simulink model "Simulation_Block_Diagram_Performance"  (R2015b)
settings: Solver=ode1  StartTime=0.0  StopTime=1200  FixedStep=0.1  RelTol=1e-3
undefined symbols (not defined in the file): udds
settings Model: Creator=wasynczu  LastModifiedBy=Kane Chew
settings DataIOCC: LimitDataPoints=off
settings DebuggingCC: ParameterUnderflowMsg=error

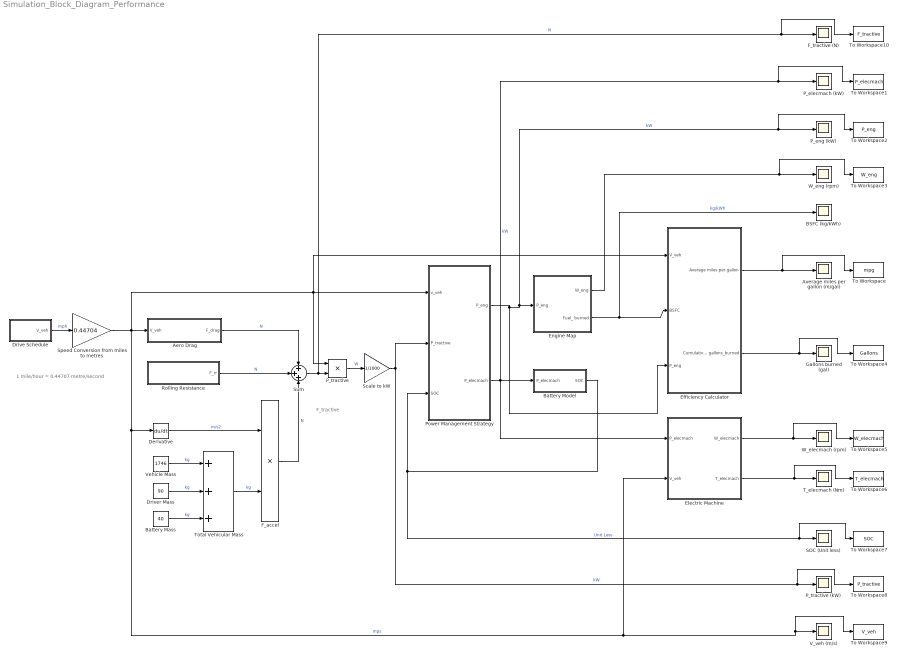
== system Simulation_Block_Diagram_Performance ==
  note: F_tractive
  note: 1 mile/hour = 0.44707 metre/second
  Aero Drag : Subsystem
  Average miles per gallon (m/gal) : Scope
  BSFC (kg/kWh) : Scope
  Battery Mass : Constant  Value=40
  "Battery Model " : Subsystem
  Derivative : Derivative
  "Drive Schedule " : Subsystem
  Driver Mass : Constant  Value=90
  Efficiency Calculator : Subsystem
  Electric Machine : Subsystem
  Engine Map : Subsystem
  F_accel : Product
  F_tractive (N) : Scope
  Gallons burned (gal) : Scope
  P_elecmach (kW) : Scope
  P_eng (kW) : Scope
  P_tractive : Product  Inputs=**
  P_tractive (kW) : Scope
  Power Management Strategy : MATLAB Function  TreatAsAtomicUnit=on
  Rolling Resistance : Subsystem
  SOC (Unit less) : Scope
  Scale to kW : Gain  Gain=1/1000
  Speed Conversion from miles to metres : Gain  Gain=0.44704
  Sum : Sum  Inputs=+++
  T_elecmach (Nm) : Scope
  To Workspace : ToWorkspace  VariableName=mpg  SaveFormat=Timeseries  SampleTime=-1
  To Workspace1 : ToWorkspace  VariableName=P_elecmach  SaveFormat=Timeseries  SampleTime=-1
  To Workspace10 : ToWorkspace  VariableName=F_tractive  SaveFormat=Timeseries  SampleTime=-1
  To Workspace2 : ToWorkspace  VariableName=P_eng  SaveFormat=Timeseries  SampleTime=-1
  To Workspace3 : ToWorkspace  VariableName=W_eng  SaveFormat=Timeseries  SampleTime=-1
  To Workspace4 : ToWorkspace  VariableName=Gallons  SaveFormat=Timeseries  SampleTime=-1
  To Workspace5 : ToWorkspace  VariableName=W_elecmach  SaveFormat=Timeseries  SampleTime=-1
  To Workspace6 : ToWorkspace  VariableName=T_elecmach  SaveFormat=Timeseries  SampleTime=-1
  To Workspace7 : ToWorkspace  VariableName=SOC  SaveFormat=Timeseries  SampleTime=-1
  To Workspace8 : ToWorkspace  VariableName=P_tractive  SaveFormat=Timeseries  SampleTime=-1
  To Workspace9 : ToWorkspace  VariableName=V_veh  SaveFormat=Timeseries  SampleTime=-1
  Total Vehicular Mass : Sum  Inputs=+++
  V_veh (m/s) : Scope
  Vehicle Mass : Constant  Value=1746
  W_elecmach (rpm) : Scope
  "W_eng (rpm) " : Scope
  wires:
  Speed Conversion from miles to metres/1 -> Electric Machine/2("V_veh "), To Workspace9/1, V_veh (m/s)/1, Derivative/1, Efficiency Calculator/1("V_veh "), Power Management Strategy/1(v_veh), P_tractive/1, Aero Drag/1(V_veh)  "mps"
  Derivative/1 -> F_accel/1  "m/s2"
  Aero Drag/1("F_drag ") -> Sum/1  "N"
  Rolling Resistance/1("F_rr ") -> Sum/2  "N"
  Sum/1 -> To Workspace10/1, F_tractive (N)/1, P_tractive/2  "N"
  P_tractive/1 -> Scale to kW/1  "W"
  Power Management Strategy/1(P_eng) -> Efficiency Calculator/3("P_eng "), To Workspace2/1, P_eng (kW)/1, Engine Map/1(P_eng)  "kW"
  "Drive Schedule "/1("V_veh ") -> Speed Conversion from miles to metres/1  "mph"
  Power Management Strategy/2(P_elecmach) -> Electric Machine/1(P_elecmach), To Workspace1/1, P_elecmach (kW)/1, "Battery Model "/1(P_elecmach)  "kW"
  "Battery Model "/1(SOC) -> Power Management Strategy/3(SOC), To Workspace7/1, SOC (Unit less)/1  "Unit Less"
  Engine Map/2(Fuel_ burned) -> BSFC (kg/kWh)/1, Efficiency Calculator/2(BSFC)  "kg/kWh"
  Engine Map/1(W_eng) -> To Workspace3/1, "W_eng (rpm) "/1
  Scale to kW/1 -> To Workspace8/1, P_tractive (kW)/1, Power Management Strategy/2(P_tractive)  "kW"
  Efficiency Calculator/1(Average miles per gallon) -> To Workspace/1, Average miles per gallon (m/gal)/1
  Efficiency Calculator/2(Cumulative gallons_burned) -> To Workspace4/1, Gallons burned (gal)/1
  Battery Mass/1 -> Total Vehicular Mass/3  "kg"
  Driver Mass/1 -> Total Vehicular Mass/2  "kg"
  Vehicle Mass/1 -> Total Vehicular Mass/1  "kg"
  Total Vehicular Mass/1 -> F_accel/2  "kg"
  F_accel/1 -> Sum/3  "N"
  Electric Machine/1(W_elecmach) -> To Workspace5/1, W_elecmach (rpm)/1
  Electric Machine/2(T_elecmach) -> To Workspace6/1, T_elecmach (Nm)/1

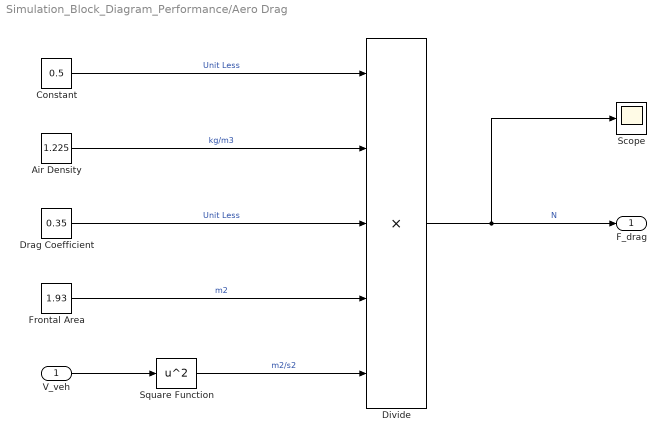
== system Simulation_Block_Diagram_Performance/Aero Drag ==
  V_veh : Inport
  Air Density : Constant  Value=1.225
  Constant : Constant  Value=0.5
  Divide : Product  Inputs=*****
  Drag Coefficient : Constant  Value=0.35
  Frontal Area : Constant  Value=1.93
  Scope : Scope
  Square Function : Math  Operator=square  SaturateOnIntegerOverflow=on
  "F_drag " : Outport
  wires:
  Divide/1 -> Scope/1, "F_drag "/1  "N"
  Air Density/1 -> Divide/2  "kg/m3"
  V_veh/1 -> Square Function/1
  Constant/1 -> Divide/1  "Unit Less"
  Frontal Area/1 -> Divide/4  "m2"
  Drag Coefficient/1 -> Divide/3  "Unit Less"
  Square Function/1 -> Divide/5  "m2/s2"

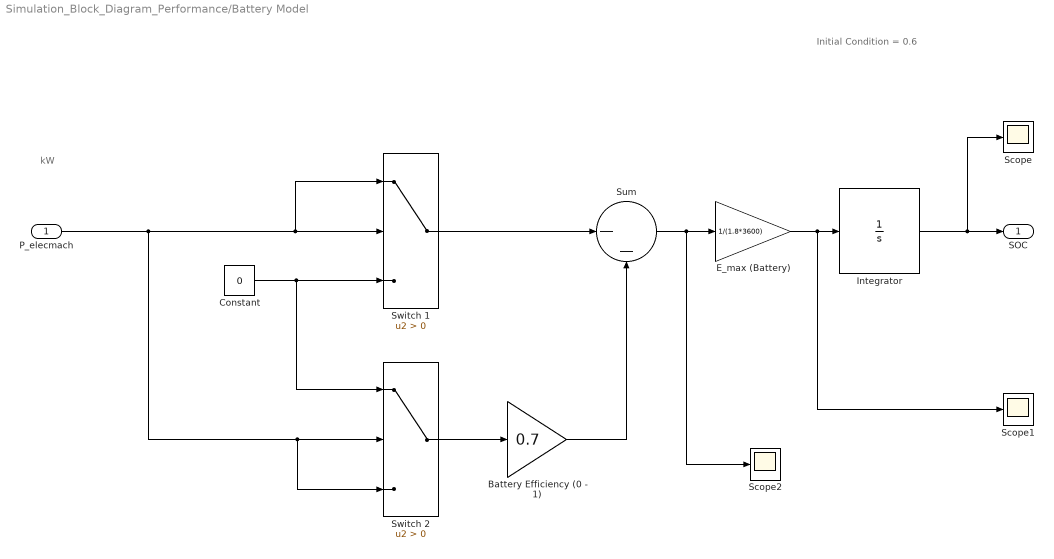
== system Simulation_Block_Diagram_Performance/Battery Model  ==
  note: kW
  note: Initial Condition = 0.6
  P_elecmach : Inport
  Battery Efficiency (0 - 1) : Gain  Gain=0.7
  Constant : Constant  Value=0
  E_max (Battery) : Gain  Gain=1/(1.8*3600)
  Integrator : Integrator  InitialCondition=0.6
  Scope : Scope
  Scope1 : Scope
  Scope2 : Scope
  Sum : Sum  Inputs=|--
  Switch 1 : Switch  Criteria=u2 > Threshold
  Switch 2 : Switch  Criteria=u2 > Threshold
  SOC : Outport
  wires:
  P_elecmach/1 -> Switch 2/3, Switch 2/2, Switch 1/1, Switch 1/2
  Constant/1 -> Switch 2/1, Switch 1/3
  Switch 1/1 -> Sum/1
  Switch 2/1 -> Battery Efficiency (0 - 1)/1
  Battery Efficiency (0 - 1)/1 -> Sum/2
  Sum/1 -> E_max (Battery)/1, Scope2/1
  E_max (Battery)/1 -> Scope1/1, Integrator/1
  Integrator/1 -> Scope/1, SOC/1

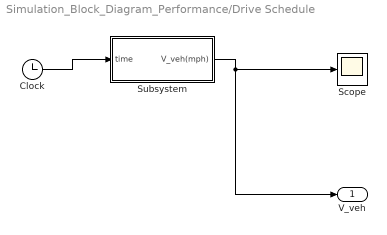
== system Simulation_Block_Diagram_Performance/Drive Schedule  ==
  Clock : Clock
  Scope : Scope
  Subsystem : Subsystem  mask{schedule=udds}
      mask prompts: schedule "drive schedule"
      mask init:
      | N=length(schedule(:,1))
  "V_veh " : Outport
  wires:
  Clock/1 -> Subsystem/1(time)
  Subsystem/1(V_veh(mph)) -> "V_veh "/1, Scope/1

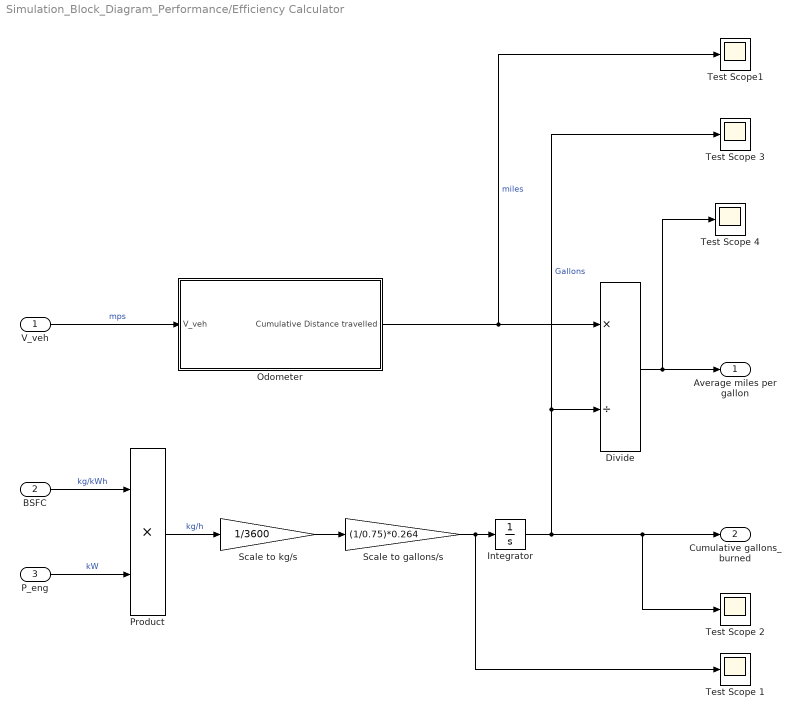
== system Simulation_Block_Diagram_Performance/Efficiency Calculator ==
  "V_veh " : Inport
  BSFC : Inport  Port=2
  "P_eng " : Inport  Port=3
  Divide : Product  Inputs=*/
  Integrator : Integrator  InitialCondition=0.001
  "Odometer " : Subsystem
  Product : Product
  Scale to gallons/s : Gain  Gain=(1/0.75)*0.264
  Scale to kg/s : Gain  Gain=1/3600
  Test Scope {1..4} (4 alike) : Scope
  Test Scope1 : Scope
  Average miles per gallon : Outport
  Cumulative gallons_burned : Outport  Port=2
  wires:
  Integrator/1 -> Divide/2, Test Scope 3/1, Test Scope 2/1, Cumulative gallons_burned/1  "Gallons"
  "V_veh "/1 -> "Odometer "/1(V_veh)  "mps"
  "Odometer "/1(Cumulative Distance travelled) -> Test Scope1/1, Divide/1  "miles"
  Divide/1 -> Test Scope 4/1, Average miles per gallon/1
  Product/1 -> Scale to kg/s/1  "kg/h"
  BSFC/1 -> Product/1  "kg/kWh"
  "P_eng "/1 -> Product/2  "kW"
  Scale to kg/s/1 -> Scale to gallons/s/1
  Scale to gallons/s/1 -> Test Scope 1/1, Integrator/1

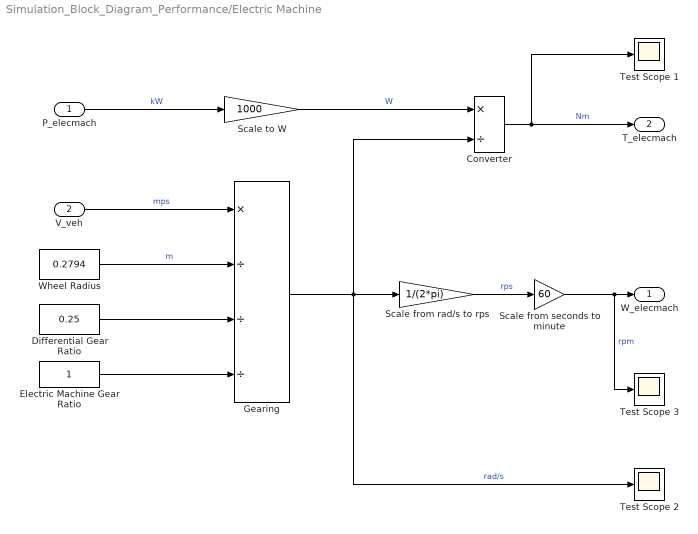
== system Simulation_Block_Diagram_Performance/Electric Machine ==
  P_elecmach : Inport
  "V_veh " : Inport  Port=2
  Converter : Product  Inputs=*/
  Differential Gear Ratio : Constant  Value=0.25
  Electric Machine Gear Ratio : Constant
  Gearing : Product  Inputs=*///
  Scale from rad/s to rps : Gain  Gain=1/(2*pi)
  Scale from seconds to minute : Gain  Gain=60
  Scale to W : Gain  Gain=1000
  Test Scope 1 : Scope
  Test Scope 2 : Scope
  Test Scope 3 : Scope
  Wheel Radius : Constant  Value=0.2794
  W_elecmach : Outport
  T_elecmach : Outport  Port=2
  wires:
  Gearing/1 -> Scale from rad/s to rps/1, Converter/2, Test Scope 2/1  "rad/s"
  Wheel Radius/1 -> Gearing/2  "m"
  Differential Gear Ratio/1 -> Gearing/3
  Electric Machine Gear Ratio/1 -> Gearing/4
  Converter/1 -> Test Scope 1/1, T_elecmach/1  "Nm"
  "V_veh "/1 -> Gearing/1  "mps"
  Scale from seconds to minute/1 -> Test Scope 3/1, W_elecmach/1  "rpm"
  P_elecmach/1 -> Scale to W/1  "kW"
  Scale to W/1 -> Converter/1  "W"
  Scale from rad/s to rps/1 -> Scale from seconds to minute/1  "rps"

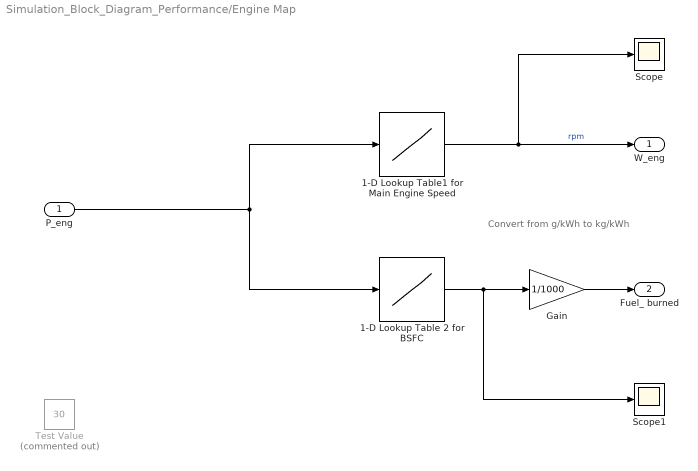
== system Simulation_Block_Diagram_Performance/Engine Map ==
  note: Convert from g/kWh to kg/kWh
  P_eng : Inport
  "1-D Lookup Table 2 for BSFC " : Lookup_n-D  NumberOfTableDimensions=1  BreakpointsForDimension1=[7,12,24,35,47,57,77,82,85]  BreakpointsForDimension2=[7,12,24,35,47]  Table=[500,400,320,285,265,255,255,265,285]  InternalRulePriority=Speed  RndMeth=Simplest  InputSameDT=on
  1-D Lookup Table1 for Main Engine Speed : Lookup_n-D  NumberOfTableDimensions=1  BreakpointsForDimension1=[7,12,24,35,47,57,77,82,85]  BreakpointsForDimension2=[7,12,24,35,47]  Table=[1009,1183,1588,1936,2318,2612,3371,3685,4014]  InternalRulePriority=Speed  RndMeth=Simplest  InputSameDT=on
  Gain : Gain  Gain=1/1000
  Scope : Scope
  Scope1 : Scope
  Test Value : Constant  Commented=on  Value=30
  W_eng : Outport
  Fuel_ burned : Outport  Port=2
  wires:
  1-D Lookup Table1 for Main Engine Speed/1 -> Scope/1, W_eng/1  "rpm"
  "1-D Lookup Table 2 for BSFC "/1 -> Scope1/1, Gain/1
  P_eng/1 -> "1-D Lookup Table 2 for BSFC "/1, 1-D Lookup Table1 for Main Engine Speed/1
  Gain/1 -> Fuel_ burned/1

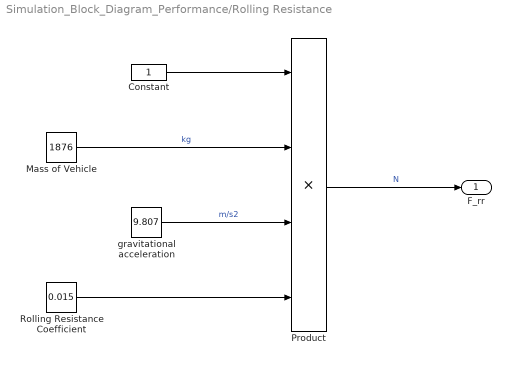
== system Simulation_Block_Diagram_Performance/Rolling Resistance ==
  Constant : Constant
  Mass of Vehicle : Constant  Value=1876
  "Product " : Product  Inputs=****
  Rolling Resistance Coefficient : Constant  Value=0.015
  "gravitational acceleration " : Constant  Value=9.807
  "F_rr " : Outport
  wires:
  Constant/1 -> "Product "/1
  "Product "/1 -> "F_rr "/1  "N"
  Mass of Vehicle/1 -> "Product "/2  "kg"
  Rolling Resistance Coefficient/1 -> "Product "/4
  "gravitational acceleration "/1 -> "Product "/3  "m/s2"

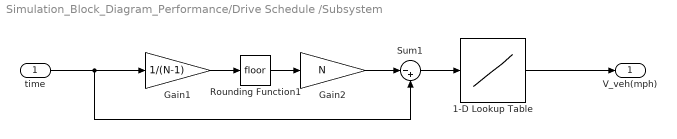
== system Simulation_Block_Diagram_Performance/Drive Schedule /Subsystem ==
  time : Inport
  1-D Lookup Table : Lookup_n-D  NumberOfTableDimensions=1  BreakpointsForDimension1=schedule(:,1)  Table=schedule(:,2)  InternalRulePriority=Speed  RndMeth=Simplest  InputSameDT=on
  Gain1 : Gain  Gain=1/(N-1)
  Gain2 : Gain  Gain=N
  Rounding Function1 : Rounding
  Sum1 : Sum  Inputs=|-+
  V_veh(mph) : Outport
  wires:
  Gain1/1 -> Rounding Function1/1
  Rounding Function1/1 -> Gain2/1
  Gain2/1 -> Sum1/1
  Sum1/1 -> 1-D Lookup Table/1
  time/1 -> Sum1/2, Gain1/1
  1-D Lookup Table/1 -> V_veh(mph)/1

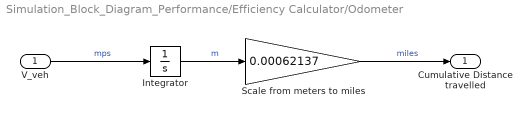
== system Simulation_Block_Diagram_Performance/Efficiency Calculator/Odometer  ==
  V_veh : Inport
  Integrator : Integrator  InitialCondition=0.001
  Scale from meters to miles : Gain  Gain=0.00062137
  Cumulative Distance travelled : Outport
  wires:
  V_veh/1 -> Integrator/1  "mps"
  Integrator/1 -> Scale from meters to miles/1  "m"
  Scale from meters to miles/1 -> Cumulative Distance travelled/1  "miles"

== matlab function Simulation_Block_Diagram_Performance/Power Management Strategy ==
  data: v_veh input; P_tractive input; P_eng output; SOC input; P_elecmach output
function [P_eng, P_elecmach] = fcn(v_veh, P_tractive, SOC)

%define variables
P_eng_min = 10;      %kW
P_eng_max = 80;      %kW

R_wheel = 0.2794;       %m
G_diff = 0.25;          %Unit less
G_trans_min = 0.3;      %Unit less
W_eng_min = 16.6667;        %revolutions per second
Scale = 1;

% The first thing to check is whether the W_eng (Engine Speed) is below 
% its minimum level. The minimum engine speed which correspond to the 
% minimum engine power level is 1000 rpm or 16.6667 rps.
% That will correspond to around 2.2 m per second or 131 m per minute.

v_veh_min   = R_wheel * G_diff * G_trans_min * W_eng_min * 2 * pi; 
% 2.1944    = 0.2794  * 0.25   * 0.3         * 16.6667   * 2 * pi

% if v_veh < v_veh_min
%             P_eng = 0;
%             P_elecmach = P_tractive;
 
%When P_tractive = 0,   P_eng = 0
%                       P_elecmach = 0
%This means that vehicle is stationary

%When P_tractive < 0,   P_eng = 0
%                       P_elecmach = P_tractive (negative value)
%This means that vehicle is stationary

if v_veh < v_veh_min
        P_eng = 0;
        P_elecmach = P_tractive;   %P_elecmach >0 => battery is discharging
        
elseif P_tractive < 10
        P_eng = 0;
        P_elecmach = P_tractive;   %P_elecmach >0 => battery is discharging
        
elseif P_tractive > 80
        P_eng = P_eng_max;
        P_elecmach = P_tractive - P_eng_max; %P_elecmach >0 => battery is discharging

else %P_tractive > 10 && P_tractive < 80
        P_elecmach = (-1)*(P_eng_max - P_tractive)*(0.6-SOC)*Scale;  
        P_eng = P_tractive - P_elecmach;
end

return
